simulink model "twotwothree"  (Simulink 8.0)
settings: Solver=ode3  StartTime=0.01  StopTime=50  FixedStep=0.001  RelTol=1e-3
libraries: simulink x1
settings Model: Creator=TheWhitescar  LastModifiedBy=bobjer
settings OptimizationCC: ExpressionDepthLimit=128
settings DebuggingCC: MultiTaskDSMMsg=warning  MultiTaskCondExecSysMsg=none  FcnCallInpInsideContextMsg=EnableAllAsWarning  StateNameClashWarn=none
settings RTWCC: IncludeERTFirstTime=on
settings CodeAppCC: CustomSymbolStrType=$N$R$M_T  InternalIdentifier=Shortened

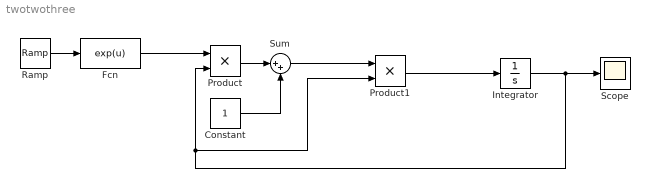
== system twotwothree ==
  Constant : Constant
  Fcn : Fcn  Expr=exp(u)
  Integrator : Integrator  InitialCondition=0.001
  Product : Product  RndMeth=Zero
  Product1 : Product  RndMeth=Zero
  Ramp : simulink/Sources/Ramp  slope=1  start=0  X0=0
  Scope : Scope
      settings: TimeRange=10  YMin=-2  YMax=1
  Sum : Sum  Inputs=|++
  wires:
  Product1/1 -> Integrator/1
  Integrator/1 -> Scope/1, Product1/2, Product/2
  Ramp/1 -> Fcn/1
  Fcn/1 -> Product/1
  Product/1 -> Sum/1
  Sum/1 -> Product1/1
  Constant/1 -> Sum/2
